simulink model "controller"  (R2018b)
settings: Solver=FixedStepAuto  StartTime=0.0  StopTime=20  FixedStep=1/100  RelTol=1e-3
libraries: simulink_extras x4
settings Model: Creator=pthb3  LastModifiedBy=pthb3

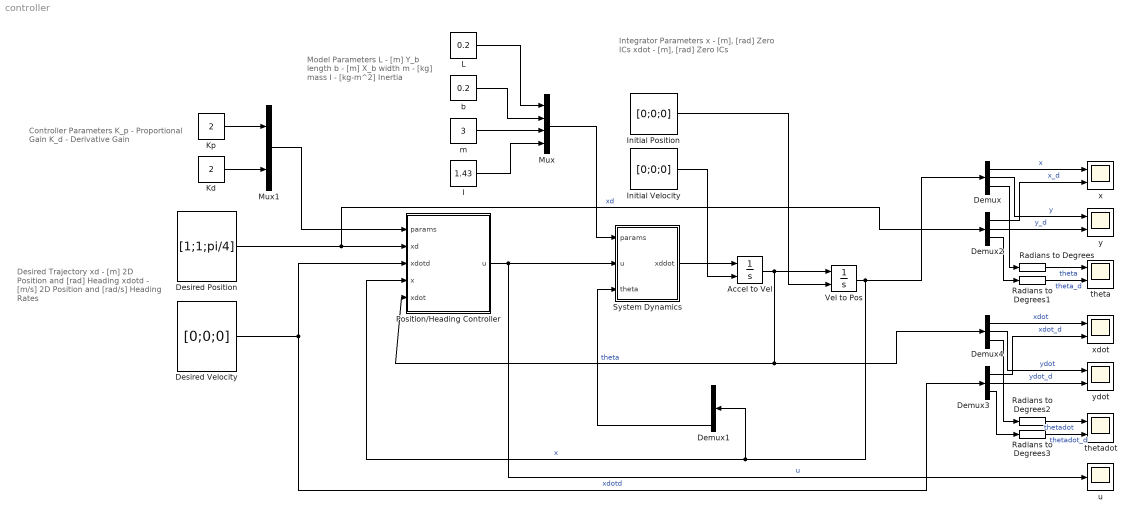
== system controller ==
  note: Model Parameters
      | L - [m] Y_b length
      | b - [m] X_b width
      | m - [kg] mass
      | I - [kg-m^2] Inertia
  note: Controller Parameters
      | K_p - Proportional Gain
      | K_d - Derivative Gain
  note: Desired Trajectory
      | xd - [m] 2D Position and
      | [rad] Heading
      | xdotd - [m/s] 2D Position and
      | [rad/s] Heading Rates
  note: Integrator Parameters
      | x - [m], [rad] Zero ICs
      | xdot - [m], [rad] Zero ICs
  Accel to Vel : Integrator  InitialConditionSource=external  InitialCondition=[0;0;0]
  Demux{,1..4} (5 alike) : Demux  Outputs=3
  Desired Position : Constant  Value=[1;1;pi/4]  VectorParams1D=off
  Desired Velocity : Constant  Value=[0;0;0]  VectorParams1D=off
  I : Constant  Value=1.43
  Initial Position : Constant  Value=[0;0;0]  VectorParams1D=off
  Initial Velocity : Constant  Value=[0;0;0]  VectorParams1D=off
  Kd : Constant  Value=2
  Kp : Constant  Value=2
  L : Constant  Value=0.2
  Mux : Mux
  Mux1 : Mux  Inputs=2
  Position/Heading Controller : MATLAB Function  TreatAsAtomicUnit=on
  Radians to Degrees{,1..3} (4 alike) : simulink_extras/Transformations/Radians to Degrees
  System Dynamics : MATLAB Function  TreatAsAtomicUnit=on
  Vel to Pos : Integrator  InitialConditionSource=external  InitialCondition=[0;0;0]
  b : Constant  Value=0.2
  m : Constant  Value=3
  theta : Scope  NumInputPorts=2
  thetadot : Scope  NumInputPorts=2
  u : Scope
  x : Scope  NumInputPorts=2
  xdot : Scope  NumInputPorts=2
  y : Scope  NumInputPorts=2
  ydot : Scope  NumInputPorts=2
  wires:
  Desired Position/1 -> Position/Heading Controller/2(xd), Demux2/1  "xd"
  Position/Heading Controller/1(u) -> System Dynamics/2(u), u/1  "u"
  System Dynamics/1(xddot) -> Accel to Vel/1
  Accel to Vel/1 -> Vel to Pos/1, Position/Heading Controller/5(xdot), Demux4/1
  Vel to Pos/1 -> Position/Heading Controller/4(x), Demux1/1, Demux/1  "x"
  Desired Velocity/1 -> Position/Heading Controller/3(xdotd), Demux3/1  "xdotd"
  Demux/1 -> x/1  "x"
  Demux/2 -> y/1  "y"
  Demux/3 -> Radians to Degrees/1
  Demux2/1 -> x/2  "x_d"
  Demux2/2 -> y/2  "y_d"
  Demux2/3 -> Radians to Degrees1/1
  Demux1/3 -> System Dynamics/3(theta)  "theta"
  Demux4/3 -> Radians to Degrees2/1
  Demux4/2 -> ydot/1  "ydot"
  Demux4/1 -> xdot/1  "xdot"
  Demux3/3 -> Radians to Degrees3/1
  Demux3/2 -> ydot/2  "ydot_d"
  Demux3/1 -> xdot/2  "xdot_d"
  Initial Position/1 -> Vel to Pos/2
  Initial Velocity/1 -> Accel to Vel/2
  L/1 -> Mux/1
  b/1 -> Mux/2
  m/1 -> Mux/3
  I/1 -> Mux/4
  Mux/1 -> System Dynamics/1(params)
  Kd/1 -> Mux1/2
  Kp/1 -> Mux1/1
  Mux1/1 -> Position/Heading Controller/1(params)
  Radians to Degrees/1 -> theta/1  "theta"
  Radians to Degrees1/1 -> theta/2  "theta_d"
  Radians to Degrees2/1 -> thetadot/1  "thetadot"
  Radians to Degrees3/1 -> thetadot/2  "thetadot_d"

== matlab function controller/Position//Heading Controller ==
  data: params input; xd input; xdotd input; u output; x input; xdot input
function u = controller(params,xd,xdotd,x,xdot)

Kp = params(1)*eye(3);
Kd = params(2)*eye(3);

u = zeros(3,1);

u = (-Kd * (xdot - xdotd)) + (-Kp * (x - xd));

== matlab function controller/System Dynamics ==
  data: params input; u input; xddot output; theta input
function xddot  = plant(params, u, theta)
    L = params(1);
    b = params(2); 
    m = params(3);
    I = params(4);
    
    H = [
        -1 -1 0 0 1 1 0 0; 
        0 0 -1 -1 0 0 1 1;
        -L L -b b -L L -b b];

    T = [
        cos(theta)/m, sin(theta)/m, 0;
        -sin(theta)/m, cos(theta)/m, 0;
        0, 0, 1/(2*I)];
    
    F = H'*inv(H*H')*inv(T)*u;
    
    xddot = T*H*F;
end
